simulink model "Exemple_Stateflow"  (R2016b)
settings: Solver=VariableStepAuto  StartTime=0.0  StopTime=inf  RelTol=1e-3
settings Model: Creator=rcostado  LastModifiedBy=rcostado

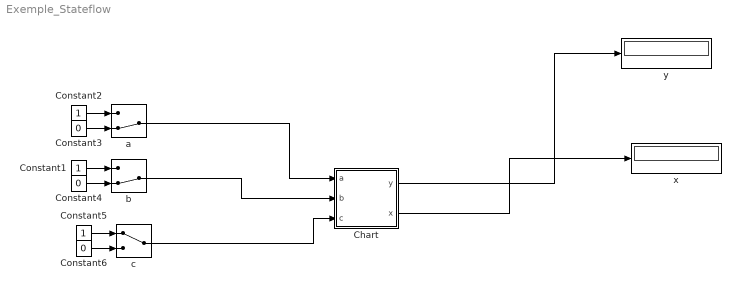
== system Exemple_Stateflow ==
  Chart : Stateflow chart  TreatAsAtomicUnit=on
  Constant1 : Constant  OutDataTypeStr=boolean
  Constant2 : Constant  OutDataTypeStr=boolean
  Constant3 : Constant  Value=0  OutDataTypeStr=boolean
  Constant4 : Constant  Value=0  OutDataTypeStr=boolean
  Constant5 : Constant  OutDataTypeStr=boolean
  Constant6 : Constant  Value=0  OutDataTypeStr=boolean
  a : ManualSwitch  CurrentSetting=0
  b : ManualSwitch  CurrentSetting=0
  c : ManualSwitch
  x : Display
  y : Display
  wires:
  a/1 -> Chart/1(a)
  Constant3/1 -> a/2
  Constant2/1 -> a/1
  b/1 -> Chart/2(b)
  Constant4/1 -> b/2
  Constant1/1 -> b/1
  Chart/1(y) -> y/1
  Chart/2(x) -> x/1
  c/1 -> Chart/3(c)
  Constant6/1 -> c/2
  Constant5/1 -> c/1

== stateflow chart Exemple_Stateflow/Chart ==
  state Etat1
    entry: y=1
    x=0
  state Etat2
    entry: y=2
  state Etat3
    entry: y=3
    state Etat4
      entry: x=1
    state Etat5
      entry: x=2
    (default) -> Etat4
    Etat5 -> Etat4 : [c==0]
    Etat4 -> Etat5 : [c==1]
  (default) -> Etat1
  Etat1 -> Etat2 : [a==1 && b==0]
  Etat2 -> Etat3 : [b==1 && a==1]
  Etat3 -> Etat1 : [a==0 && b==0]
  data: y output; a input; b input; c input; x output
